simulink model "controller_angular_rate_pitch"  (R2019b)
settings: Solver=FixedStepAuto  StartTime=0.0  StopTime=10.0  FixedStep=1/sim_freq  RelTol=1e-3
undefined symbols (not defined in the file): body_rates_dterm_cutoff, body_rates_filter_denom, body_rates_filter_num, DiscIntNeverNeededParam, G_PR_OL_DENOM, G_PR_OL_NUM, K_qd, K_qi, K_qp, q_int_lim, q_max
libraries: simulink x2
settings Model: Creator=francois  LastModifiedBy=francois

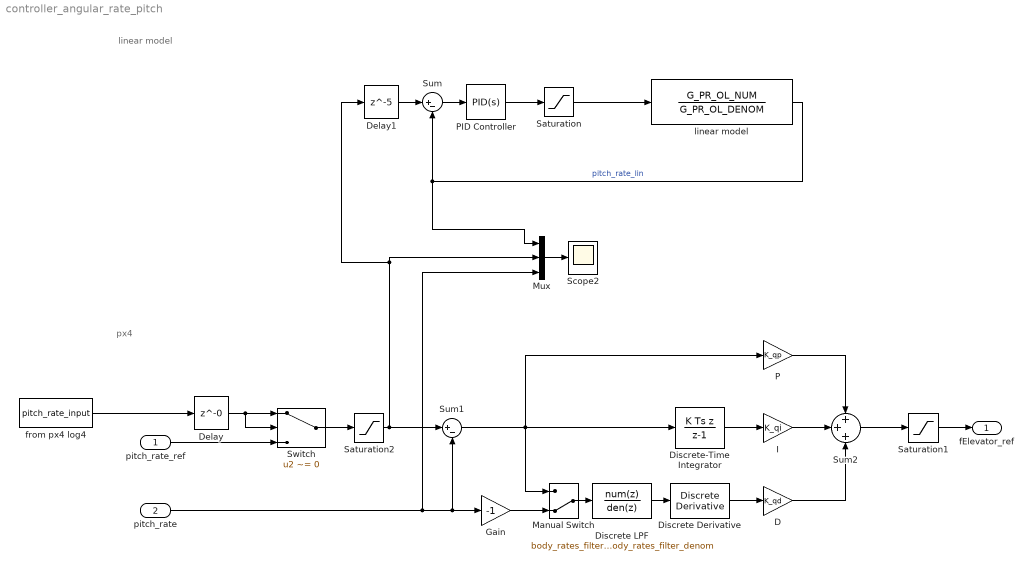
== system controller_angular_rate_pitch ==
  note: px4
  note: linear model
  pitch_rate_ref : Inport
  pitch_rate : Inport  Port=2
  D : Gain  Gain=K_qd
  Delay : Delay  DelayLength=0
  Delay1 : Delay  DelayLength=5
  Discrete Derivative : simulink/Discrete/Discrete Derivative  gainval=1.0  ICPrevScaledInput=0.0  OutMin=[]  OutMax=[]  OutDataType=fixdt(1, 16)  OutScaling=2^-10  DoSatur=off
  Discrete LPF : DiscreteTransferFcn  Numerator=body_rates_filter_num  Denominator=body_rates_filter_denom
  Discrete-Time Integrator : DiscreteIntegrator  IntegratorMethod=Integration: Backward Euler  SampleTime=-1  LimitOutput=on  UpperSaturationLimit=q_int_lim  LowerSaturationLimit=-q_int_lim  ICPrevOutput=DiscIntNeverNeededParam  ICPrevScaledInput=DiscIntNeverNeededParam
  Gain : Gain  Gain=-1
  I : Gain  Gain=K_qi
  Manual Switch : ManualSwitch  CurrentSetting=0
  Mux : Mux  Inputs=3
  P : Gain  Gain=K_qp
  "PID Controller " : simulink/Continuous/PID Controller  Controller=PID  Form=Parallel  TimeDomain=Continuous-time  SampleTime=-1  IntegratorMethod=Forward Euler  FilterMethod=Forward Euler  ControllerParametersSource=internal  P=K_qp  I=K_qi  D=K_qd  UseFilter=on  N=body_rates_dterm_cutoff*10  TunerSelectOption=Transfer Function Based (PID Tuner App)  InitialConditionSource=internal  InitialConditionForIntegrator=0  InitialConditionForFilter=0  DifferentiatorICPrevScaledInput=0  ExternalReset=none  TrackingMode=off  Kt=1  LimitOutput=off  UpperSaturationLimit=inf  LowerSaturationLimit=-inf  LinearizeAsGain=on  AntiWindupMode=none  Kb=1  POutMin=[]  POutMax=[]  IOutMin=[]  IOutMax=[]  DOutMin=[]  DOutMax=[]  NOutMin=[]  NOutMax=[]  SumOutMin=[]  SumOutMax=[]  SaturationOutMin=[]  SaturationOutMax=[]  PParamMin=[]  PParamMax=[]  IParamMin=[]  IParamMax=[]  DParamMin=[]  DParamMax=[]  NParamMin=[]  NParamMax=[]  KbParamMin=[]  KbParamMax=[]  KtParamMin=[]  KtParamMax=[]  KbOutMin=[]  KbOutMax=[]  KtOutMin=[]  KtOutMax=[]  IntegratorOutMin=[]  IntegratorOutMax=[]  FilterOutMin=[]  FilterOutMax=[]  SumI1OutMin=[]  SumI1OutMax=[]  SumI2OutMin=[]  SumI2OutMax=[]  SumI3OutMin=[]  SumI3OutMax=[]  SumI4OutMin=[]  SumI4OutMax=[]  SumDOutMin=[]  SumDOutMax=[]  DifferentiatorOutMin=[]  DifferentiatorOutMax=[]  FilterDiffOutCoefMin=[]  FilterDiffOutCoefMax=[]  ReciprocalOutMin=[]  ReciprocalOutMax=[]  SumDenOutMin=[]  SumDenOutMax=[]  SumNumOutMin=[]  SumNumOutMax=[]  DivideOutMin=[]  DivideOutMax=[]  IntegratorContinuousStateAttributes=''  IntegratorStateMustResolveToSignalObject=off  IntegratorRTWStateStorageClass=Auto  FilterContinuousStateAttributes=''  FilterStateMustResolveToSignalObject=off  FilterRTWStateStorageClass=Auto  ParallelPVariant=InternalParameters  IdealPVariant=Disabled  IVariant=InternalParameters  DVariant=InternalParameters  IntegratorVariant=Continuous  SatVariant=Disabled  AWVariant=Passthrough  PCopyVariant=Disabled  TRVariant=Disabled  FdbkBlocksVariant=Forward  IdealPFdbkVariant=Disabled  SatFdbkVariant=Disabled  DerivativeFilterVariant=ContFilter  NVariant=InternalParameters  NCopyVariant=Disabled  FilterICVariant=InternalICsFilter  IntegratorICVariant=InternalICs  ExternalResetVariant=Disabled  TRSumVariant=Passthrough  SumFdbkVariant=Disabled  SumVariant=Sum_PID
  Saturation : Saturate  UpperLimit=1  LowerLimit=-1
  Saturation1 : Saturate  UpperLimit=1  LowerLimit=-1
  Saturation2 : Saturate  UpperLimit=q_max  LowerLimit=-q_max
  Scope2 : Scope
  Sum : Sum  Inputs=|+-
  Sum1 : Sum  Inputs=|+-
  Sum2 : Sum  Inputs=+++
  Switch : Switch  Criteria=u2 ~= 0
  from px4 log4 : FromWorkspace  VariableName=pitch_rate_input  SampleTime=0
  linear model : TransferFcn  Numerator=G_PR_OL_NUM  Denominator=G_PR_OL_DENOM
  fElevator_ref : Outport
  wires:
  Sum/1 -> "PID Controller "/1
  pitch_rate_ref/1 -> Switch/3
  linear model/1 -> Mux/1, Sum/2  "pitch_rate_lin"
  Saturation/1 -> linear model/1
  "PID Controller "/1 -> Saturation/1
  Sum1/1 -> Discrete-Time Integrator/1, P/1, Manual Switch/1
  I/1 -> Sum2/2
  P/1 -> Sum2/1
  D/1 -> Sum2/3
  Discrete-Time Integrator/1 -> I/1
  Discrete Derivative/1 -> D/1
  Manual Switch/1 -> Discrete LPF/1
  Discrete LPF/1 -> Discrete Derivative/1
  Sum2/1 -> Saturation1/1
  Saturation1/1 -> fElevator_ref/1
  pitch_rate/1 -> Mux/3, Sum1/2, Gain/1
  Gain/1 -> Manual Switch/2
  Saturation2/1 -> Sum1/1, Mux/2, Delay1/1
  Switch/1 -> Saturation2/1
  Delay/1 -> Switch/2, Switch/1
  from px4 log4/1 -> Delay/1
  Delay1/1 -> Sum/1
  Mux/1 -> Scope2/1
